simulink model "Final"  (R2025b)
settings: Solver=ode4  StartTime=0.0  StopTime=3  FixedStep=1e-5  RelTol=1e-3
values from neighbouring files (symbols this model uses):
  BAT_A = BAT    [simulink_init_params_CORRECTED.m]
  BAT_B = BAT    [simulink_init_params_CORRECTED.m]
  omega_init_cmd = SpeedRef_rpm_cmd * 2 * pi / 60    (= 314.159265359)    [simulink_init_params_CORRECTED.m]
  SpeedRef_rpm_cmd = 3000    [simulink_init_params_CORRECTED.m]
  TorqueRef_gen_Nm_cmd = -100    [simulink_init_params_CORRECTED.m]
undefined symbols (not defined in the file or in its folder): BAT, DCDC, DCLINK, FOC, FW, INV, MECH, PMSM, THERM
libraries: slpidlib x6, mcbcontrolslib x2
(part 1 of 2)
settings Model: Creator=barne  LastModifiedBy=barne

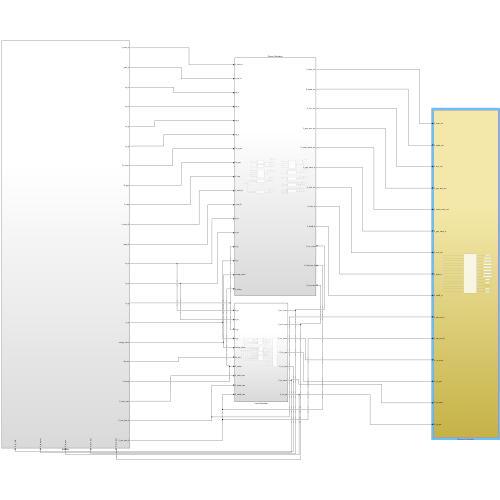
[thumbnail: Simulink's stored preview of the top-level diagram]
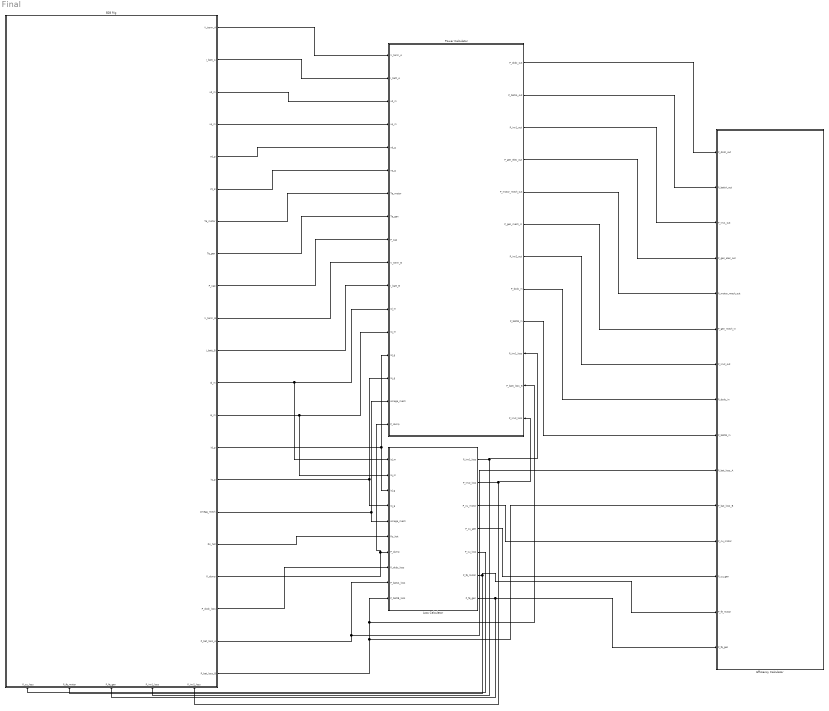
== system Final ==
  "B2B Rig " : Subsystem
      settings: PortSchema="{\"entries\":[{\"content\":{\"sides\":[{\"content\":{},\"type\":\"ConnectorPlacement.EquallySpacedRectSide\",\"uuid\":\"35d57d76-af41-41f5-b20d-811f83701aa2\"},{\"content\":{\"connectorIds\":[\"Out1\",\"Out2\",\"Out3\",\"Out4\",\"Out5\",\"Out6\",\"Out7\",\"Out8\",\"Out9\",\"Out10\",\"Out11\",\"Out12\",\"Out13\",\"Out14\",\"Out15\",\"Out16\",\"Out17\",\"Out18\",\"Out19\",\"Out20\",\"Out21\"],\"side\":\"RIGHT\"},\"type\":\"ConnectorPlacement.EquallySpacedRectSide\",\"uuid\":\"9a3983e4-5d9f-4748-b79f-80b2f2f1c763\"},{\"content\":{\"side\":\"TOP\"},\"type\":\"ConnectorPlacement.EquallySpacedRectSide\",\"uuid\":\"9f326ba3-25e1-42ff-85bf-75e4830b2979\"},{\"content\":{\"connectorIds\":[\"In1\",\"In2\",\"In3\",\"In4\",\"In5\"],\"side\":\"BOTTOM\"},\"type\":\"ConnectorPlacement.EquallySpacedRectSide\",\"uuid\":\"a03ba88c-9183-421b-aa71-4f6f8afbf457\"}]},\"type\":\"ConnectorPlacement.EquallySpacedConnector\",\"uuid\":\"4b320d25-9064-42a3-b743-e8ce904cf471\"}],\"packageUris\":[\"http://schema.mathworks.com/mf0/Connector/R2020b\"],\"version\":\"1.0\"}"
  Efficiency Calculator : Subsystem
  Loss Calculator : Subsystem
  Power Calculator : Subsystem
      settings: PortSchema="{\"entries\":[{\"content\":{\"sides\":[{\"content\":{\"connectorIds\":[\"In1\",\"In2\",\"In3\",\"In4\",\"In5\",\"In6\",\"In7\",\"In8\",\"In9\",\"In10\",\"In11\",\"In12\",\"In13\",\"In14\",\"In15\",\"In16\",\"In17\"]},\"type\":\"ConnectorPlacement.EquallySpacedRectSide\",\"uuid\":\"b3a63054-6e96-48ec-b2cd-405618c65b15\"},{\"content\":{\"connectorIds\":[\"Out1\",\"Out2\",\"Out3\",\"Out4\",\"Out5\",\"Out6\",\"Out7\",\"Out8\",\"Out9\",\"In18\",\"In19\",\"In20\"],\"side\":\"RIGHT\"},\"type\":\"ConnectorPlacement.EquallySpacedRectSide\",\"uuid\":\"702f6dd8-defa-44ea-83b1-91536885574a\"},{\"content\":{\"side\":\"TOP\"},\"type\":\"ConnectorPlacement.EquallySpacedRectSide\",\"uuid\":\"42970328-246a-4ab1-891c-aefddd02ac7d\"}]},\"type\":\"ConnectorPlacement.EquallySpacedConnector\",\"uuid\":\"4be053d2-cc40-44fc-9305-e73801c5c4b1\"}],\"packageUris\":[\"http://schema.mathworks.com/mf0/Connector/R2020b\"],\"version\":\"1.0\"}"
  wires:
  "B2B Rig "/20(P_bat_loss_A) -> Loss Calculator/9(P_battA_loss), Efficiency Calculator/10(P_bat_loss_A)
  "B2B Rig "/1(V_term_A) -> Power Calculator/1(V_term_A)
  "B2B Rig "/7(Te_motor) -> Power Calculator/7(Te_motor)
  Power Calculator/6(P_gen_mech_in) -> Efficiency Calculator/6(P_gen_mech_in)
  "B2B Rig "/19(P_dcdc_loss) -> Loss Calculator/8(P_dcdc_loss)
  "B2B Rig "/2(I_batt_A) -> Power Calculator/2(I_batt_A)
  "B2B Rig "/3(vd_m) -> Power Calculator/3("vd_m ")
  "B2B Rig "/8(Te_gen) -> Power Calculator/8(Te_gen)
  "B2B Rig "/6(vq_g) -> Power Calculator/6(vq_g)
  "B2B Rig "/4(vq_m) -> Power Calculator/4(vq_m)
  "B2B Rig "/5(vd_g) -> Power Calculator/5(vd_g)
  "B2B Rig "/10(V_term_B) -> Power Calculator/10(V_term_B)
  Power Calculator/9(P_battB_in) -> Efficiency Calculator/9(P_battB_in)
  "B2B Rig "/11(I_batt_B) -> Power Calculator/11(I_batt_B)
  "B2B Rig "/12(id_m) -> Power Calculator/12(id_m), Loss Calculator/1(id_m)
  "B2B Rig "/13(iq_m) -> Power Calculator/13(iq_m), Loss Calculator/2(iq_m)
  "B2B Rig "/14(id_g) -> Power Calculator/14(id_g), Loss Calculator/3(id_g)
  Loss Calculator/1(P_inv1_loss) -> Power Calculator/18(P_inv1_loss), "B2B Rig "/4(P_inv1_loss)
  "B2B Rig "/15(iq_g) -> Power Calculator/15(iq_g), Loss Calculator/4(iq_g)
  "B2B Rig "/16(omega_mech) -> Power Calculator/16(omega_mech), Loss Calculator/5(omega_mech)
  Power Calculator/8(P_dcdc_in) -> Efficiency Calculator/8(P_dcdc_in)
  Power Calculator/4(P_gen_elec_out) -> Efficiency Calculator/4(P_gen_elec_out)
  "B2B Rig "/17(Rs_hot) -> Loss Calculator/6(Rs_hot)
  "B2B Rig "/18(P_dump) -> Power Calculator/17(P_dump), Loss Calculator/7(P_dump)
  "B2B Rig "/21(P_bat_loss_B) -> Loss Calculator/10(P_battB_loss), Power Calculator/19(P_batt_loss_B), Efficiency Calculator/11(P_bat_loss_B)
  Power Calculator/2(P_battA_out) -> Efficiency Calculator/2(P_battA_out)
  Power Calculator/3(P_inv1_out) -> Efficiency Calculator/3(P_inv1_out)
  Power Calculator/5(P_motor_mech_out) -> Efficiency Calculator/5(P_motor_mech_out)
  Power Calculator/7(P_inv2_out) -> Efficiency Calculator/7(P_inv2_out)
  Power Calculator/1(P_dcdc_out) -> Efficiency Calculator/1(P_dcdc_out)
  "B2B Rig "/9(P_cap) -> Power Calculator/9(P_cap)
  Loss Calculator/2(P_inv2_loss) -> Power Calculator/20(P_inv2_loss), "B2B Rig "/5(P_inv2_loss)
  Loss Calculator/5(P_cu_loss) -> "B2B Rig "/1(P_cu_loss)
  Loss Calculator/3(P_cu_motor) -> Efficiency Calculator/12(P_cu_motor)
  Loss Calculator/4(P_cu_gen) -> Efficiency Calculator/13(P_cu_gen)
  Loss Calculator/6(P_fe_motor) -> Efficiency Calculator/14(P_fe_motor), "B2B Rig "/2(P_fe_motor)
  Loss Calculator/7(P_fe_gen) -> "B2B Rig "/3(P_fe_gen), Efficiency Calculator/15(P_fe_gen)

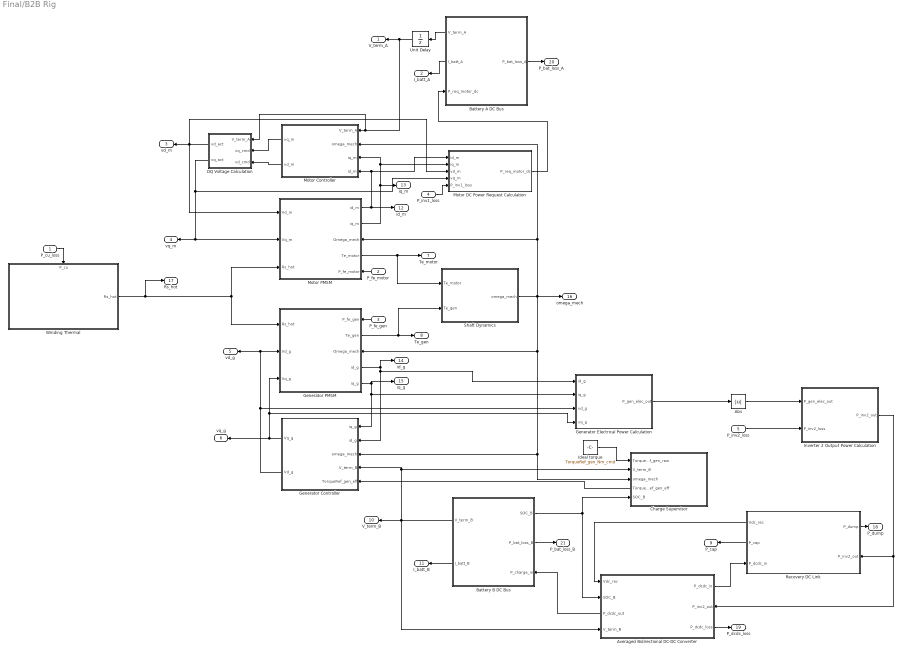
== system Final/B2B Rig  ==
  P_cu_loss : Inport
  P_fe_motor : Inport  Port=2
  P_fe_gen : Inport  Port=3
  P_inv1_loss : Inport  Port=4
  P_inv2_loss : Inport  Port=5
  Abs : Abs  SaturateOnIntegerOverflow=off
  Averaged Bidirectional DC-DC Converter : Subsystem
      settings: PortSchema="{\"entries\":[{\"content\":{\"sides\":[{\"content\":{\"connectorIds\":[\"In1\",\"In2\",\"Out3\",\"In3\"]},\"type\":\"ConnectorPlacement.EquallySpacedRectSide\",\"uuid\":\"c75c4d97-d9fe-4485-978f-a90415bcd4b0\"},{\"content\":{\"connectorIds\":[\"Out1\",\"In4\",\"Out2\"],\"side\":\"RIGHT\"},\"type\":\"ConnectorPlacement.EquallySpacedRectSide\",\"uuid\":\"ca166856-9308-4393-8aae-1a6df3904c27\"},{\"content\":{\"side\":\"TOP\"},\"type\":\"ConnectorPlacement.EquallySpacedRectSide\",\"uuid\":\"ee8baf38-1402-4df1-aabb-1ba4a360531c\"}]},\"type\":\"ConnectorPlacement.EquallySpacedConnector\",\"uuid\":\"7d2a7e48-193d-4e7a-9033-8960d9759152\"}],\"packageUris\":[\"http://schema.mathworks.com/mf0/Connector/R2020b\"],\"version\":\"1.0\"}"
  Battery A DC Bus : Subsystem
      settings: PortSchema="{\"entries\":[{\"content\":{\"sides\":[{\"content\":{\"connectorIds\":[\"Out2\",\"Out3\",\"In1\"]},\"type\":\"ConnectorPlacement.EquallySpacedRectSide\",\"uuid\":\"be2ffeb8-897f-4fb0-9a8e-cb986b650704\"},{\"content\":{\"connectorIds\":[\"Out1\"],\"side\":\"RIGHT\"},\"type\":\"ConnectorPlacement.EquallySpacedRectSide\",\"uuid\":\"a4a4824a-f919-417d-bceb-2ba105cf5ab4\"},{\"content\":{\"side\":\"TOP\"},\"type\":\"ConnectorPlacement.EquallySpacedRectSide\",\"uuid\":\"5f1b089a-09aa-462b-ad0f-8275eb166d2e\"}]},\"type\":\"ConnectorPlacement.EquallySpacedConnector\",\"uuid\":\"42065a04-5d0c-471f-9e1f-47cde4d39611\"}],\"packageUris\":[\"http://schema.mathworks.com/mf0/Connector/R2020b\"],\"version\":\"1.0\"}"
  Battery B DC Bus : Subsystem
      settings: PortSchema="{\"entries\":[{\"content\":{\"sides\":[{\"content\":{\"connectorIds\":[\"Out3\",\"Out4\"]},\"type\":\"ConnectorPlacement.EquallySpacedRectSide\",\"uuid\":\"be2ffeb8-897f-4fb0-9a8e-cb986b650704\"},{\"content\":{\"connectorIds\":[\"Out1\",\"Out2\",\"In1\"],\"side\":\"RIGHT\"},\"type\":\"ConnectorPlacement.EquallySpacedRectSide\",\"uuid\":\"a4a4824a-f919-417d-bceb-2ba105cf5ab4\"},{\"content\":{\"side\":\"TOP\"},\"type\":\"ConnectorPlacement.EquallySpacedRectSide\",\"uuid\":\"5f1b089a-09aa-462b-ad0f-8275eb166d2e\"}]},\"type\":\"ConnectorPlacement.EquallySpacedConnector\",\"uuid\":\"42065a04-5d0c-471f-9e1f-47cde4d39611\"}],\"packageUris\":[\"http://schema.mathworks.com/mf0/Connector/R2020b\"],\"version\":\"1.0\"}"
  Charge Supervisor : Subsystem
      settings: PortSchema="{\"entries\":[{\"content\":{\"sides\":[{\"content\":{\"connectorIds\":[\"In1\",\"In2\",\"In3\",\"Out1\",\"In4\"]},\"type\":\"ConnectorPlacement.EquallySpacedRectSide\",\"uuid\":\"511ba033-72f1-459a-95dc-757aaac28559\"},{\"content\":{\"side\":\"RIGHT\"},\"type\":\"ConnectorPlacement.EquallySpacedRectSide\",\"uuid\":\"14c3a67f-ee08-4dd0-a6b8-6f3110f3c251\"},{\"content\":{\"side\":\"TOP\"},\"type\":\"ConnectorPlacement.EquallySpacedRectSide\",\"uuid\":\"028d3826-294c-4b4b-bd61-9c2d945a5125\"}]},\"type\":\"ConnectorPlacement.EquallySpacedConnector\",\"uuid\":\"eacb2f62-77aa-43a8-a347-5c269c986bc2\"}],\"packageUris\":[\"http://schema.mathworks.com/mf0/Connector/R2020b\"],\"version\":\"1.0\"}"
  DQ Voltage Calculation : MATLAB Function  TreatAsAtomicUnit=on
  Generator Controller : Subsystem
  Generator Electrical Power Calculation : MATLAB Function  TreatAsAtomicUnit=on
  Generator PMSM : Subsystem
      settings: PortSchema="{\"entries\":[{\"content\":{\"sides\":[{\"content\":{\"connectorIds\":[\"In1\",\"In2\",\"In3\"]},\"type\":\"ConnectorPlacement.EquallySpacedRectSide\",\"uuid\":\"07b3d59a-f926-4a7d-ab04-b9c2d2b414a8\"},{\"content\":{\"connectorIds\":[\"In4\",\"Out1\",\"In5\",\"Out2\",\"Out3\"],\"side\":\"RIGHT\"},\"type\":\"ConnectorPlacement.EquallySpacedRectSide\",\"uuid\":\"bee2f74a-f43a-4aee-bb40-851f5cf071b9\"},{\"content\":{\"side\":\"TOP\"},\"type\":\"ConnectorPlacement.EquallySpacedRectSide\",\"uuid\":\"c59a3e1f-4ae4-432c-9c2c-e4c61d9f9d5f\"}]},\"type\":\"ConnectorPlacement.EquallySpacedConnector\",\"uuid\":\"492bf2cb-efe4-439e-9d58-c452a678f7e2\"}],\"packageUris\":[\"http://schema.mathworks.com/mf0/Connector/R2020b\"],\"version\":\"1.0\"}"
  "Ideal torque " : Constant  Value=TorqueRef_gen_Nm_cmd
  Inverter 2 Output Power Calculation : MATLAB Function  TreatAsAtomicUnit=on
  Motor Controller : Subsystem
  Motor DC Power Request Calculation : MATLAB Function  TreatAsAtomicUnit=on
  Motor PMSM : Subsystem
      settings: PortSchema="{\"entries\":[{\"content\":{\"sides\":[{\"content\":{\"connectorIds\":[\"In1\",\"In2\",\"In3\"]},\"type\":\"ConnectorPlacement.EquallySpacedRectSide\",\"uuid\":\"07b3d59a-f926-4a7d-ab04-b9c2d2b414a8\"},{\"content\":{\"connectorIds\":[\"Out1\",\"Out2\",\"In4\",\"Out3\",\"In5\"],\"side\":\"RIGHT\"},\"type\":\"ConnectorPlacement.EquallySpacedRectSide\",\"uuid\":\"bee2f74a-f43a-4aee-bb40-851f5cf071b9\"},{\"content\":{\"side\":\"TOP\"},\"type\":\"ConnectorPlacement.EquallySpacedRectSide\",\"uuid\":\"c59a3e1f-4ae4-432c-9c2c-e4c61d9f9d5f\"}]},\"type\":\"ConnectorPlacement.EquallySpacedConnector\",\"uuid\":\"492bf2cb-efe4-439e-9d58-c452a678f7e2\"}],\"packageUris\":[\"http://schema.mathworks.com/mf0/Connector/R2020b\"],\"version\":\"1.0\"}"
  Recovery DC Link : Subsystem
      settings: PortSchema="{\"entries\":[{\"content\":{\"sides\":[{\"content\":{\"connectorIds\":[\"Out2\",\"Out3\",\"In1\"]},\"type\":\"ConnectorPlacement.EquallySpacedRectSide\",\"uuid\":\"bc30b136-784e-45bb-af95-843f9a6ddb33\"},{\"content\":{\"connectorIds\":[\"Out1\",\"In2\"],\"side\":\"RIGHT\"},\"type\":\"ConnectorPlacement.EquallySpacedRectSide\",\"uuid\":\"2f565876-dfa7-4c6c-9c16-5c008dcf0872\"},{\"content\":{\"side\":\"TOP\"},\"type\":\"ConnectorPlacement.EquallySpacedRectSide\",\"uuid\":\"25b582a4-9873-4df9-8c8d-16d41c520507\"}]},\"type\":\"ConnectorPlacement.EquallySpacedConnector\",\"uuid\":\"ee427943-397a-4e08-9409-61b509181f95\"}],\"packageUris\":[\"http://schema.mathworks.com/mf0/Connector/R2020b\"],\"version\":\"1.0\"}"
  Shaft Dynamics : Subsystem
  Unit Delay : UnitDelay  InitialCondition=BAT_A.V_nom  SampleTime=FOC.Ts  HasFrameUpgradeWarning=on
  Winding Thermal : Subsystem
      settings: PortSchema="{\"entries\":[{\"content\":{\"sides\":[{\"content\":{\"connectorIds\":[\"Out1\"]},\"type\":\"ConnectorPlacement.EquallySpacedRectSide\",\"uuid\":\"4eefefd2-644d-4013-be3c-911fe82f6150\"},{\"content\":{\"side\":\"RIGHT\"},\"type\":\"ConnectorPlacement.EquallySpacedRectSide\",\"uuid\":\"de5532ad-21e1-424d-bba4-8a6bf70e2e70\"},{\"content\":{\"connectorIds\":[\"In1\"],\"side\":\"TOP\"},\"type\":\"ConnectorPlacement.EquallySpacedRectSide\",\"uuid\":\"20b811fb-5177-4825-9338-966d2d4b1cfa\"}]},\"type\":\"ConnectorPlacement.EquallySpacedConnector\",\"uuid\":\"f93ab436-6edc-4857-8a77-fc7572dced6a\"}],\"packageUris\":[\"http://schema.mathworks.com/mf0/Connector/R2020b\"],\"version\":\"1.0\"}"
  V_term_A : Outport
  I_batt_A : Outport  Port=2
  vd_m : Outport  Port=3
  vq_m : Outport  Port=4
  vd_g : Outport  Port=5
  vq_g : Outport  Port=6
  Te_motor : Outport  Port=7
  Te_gen : Outport  Port=8
  P_cap : Outport  Port=9
  V_term_B : Outport  Port=10
  I_batt_B : Outport  Port=11
  id_m : Outport  Port=12
  iq_m : Outport  Port=13
  id_g : Outport  Port=14
  iq_g : Outport  Port=15
  omega_mech : Outport  Port=16
  Rs_hot : Outport  Port=17
  P_dump : Outport  Port=18
  P_dcdc_loss : Outport  Port=19
  P_bat_loss_A : Outport  Port=20
  P_bat_loss_B : Outport  Port=21
  wires:
  Battery B DC Bus/1(SOC_B) -> Charge Supervisor/4(SOC_B), Averaged Bidirectional DC-DC Converter/2(SOC_B)
  Shaft Dynamics/1(omega_mech) -> Motor Controller/2(omega_mech), Motor PMSM/4(Omega_mech), omega_mech/1, Charge Supervisor/3(omega_mech), Generator Controller/3(omega_mech), Generator PMSM/5(Omega_mech)
  Battery B DC Bus/3(V_term_B) -> Averaged Bidirectional DC-DC Converter/3(V_term_B), V_term_B/1, Generator Controller/4(V_term_B), Charge Supervisor/2(V_term_B)
  Winding Thermal/1(Rs_hot) -> Rs_hot/1, Generator PMSM/1(Rs_hot), Motor PMSM/3(Rs_hot)
  Averaged Bidirectional DC-DC Converter/3(P_dcdc_out) -> Battery B DC Bus/1(P_charge_in)
  Motor PMSM/1(id_m) -> Motor DC Power Request Calculation/1(id_m), Motor Controller/4(id_m), id_m/1
  Generator PMSM/3(iq_g) -> iq_g/1, Generator Controller/1(iq_g), Generator Electrical Power Calculation/2(iq_g)
  Motor PMSM/2(iq_m) -> Motor Controller/3(iq_m), Motor DC Power Request Calculation/2(iq_m), iq_m/1
  Recovery DC Link/1(P_dump) -> P_dump/1
  P_cu_loss/1 -> Winding Thermal/1(P_cu)
  Recovery DC Link/2(Vdc_rec) -> Averaged Bidirectional DC-DC Converter/1(Vdc_rec)
  Battery A DC Bus/2(V_term_A) -> Unit Delay/1
  Averaged Bidirectional DC-DC Converter/1(P_dcdc_in) -> Recovery DC Link/1(P_dcdc_in)
  Generator Controller/1(Vq_g) -> Generator Electrical Power Calculation/4(vq_g), Generator PMSM/3(Vq_g), vq_g/1
  Generator Controller/2(Vd_g) -> vd_g/1, Generator PMSM/2(Vd_g), Generator Electrical Power Calculation/3(vd_g)
  Motor PMSM/3(Te_motor) -> Shaft Dynamics/1(Te_motor), Te_motor/1
  Generator PMSM/1(Te_gen) -> Shaft Dynamics/2(Te_gen), Te_gen/1
  "Ideal torque "/1 -> Charge Supervisor/1(TorqueRef_gen_raw)
  Averaged Bidirectional DC-DC Converter/2(P_dcdc_loss) -> P_dcdc_loss/1
  Battery A DC Bus/1(P_bat_loss_A) -> P_bat_loss_A/1
  Battery B DC Bus/2(P_bat_loss_B) -> P_bat_loss_B/1
  Battery B DC Bus/4(I_batt_B) -> I_batt_B/1
  Motor DC Power Request Calculation/1(P_req_motor_dc) -> Battery A DC Bus/1(P_req_motor_dc)
  Charge Supervisor/1(TorqueRef_gen_eff) -> Generator Controller/5(TorqueRef_gen_eff)
  Generator PMSM/2(id_g) -> id_g/1, Generator Electrical Power Calculation/1(id_g), Generator Controller/2(id_g)
  Generator Electrical Power Calculation/1(P_gen_elec_out) -> Abs/1
  Unit Delay/1 -> DQ Voltage Calculation/1(V_term_A), Motor Controller/1(V_term_A), V_term_A/1
  Battery A DC Bus/3(I_batt_A) -> I_batt_A/1
  P_fe_motor/1 -> Motor PMSM/5(P_fe_motor)
  Motor Controller/1(vq_m) -> DQ Voltage Calculation/2(vq_cmd)
  Motor Controller/2(vd_m) -> DQ Voltage Calculation/3(vd_cmd)
  DQ Voltage Calculation/1(vd_act) -> Motor PMSM/1(Vd_m), Motor DC Power Request Calculation/3(vd_m), vd_m/1
  DQ Voltage Calculation/2(vq_act) -> vq_m/1, Motor PMSM/2(Vq_m), Motor DC Power Request Calculation/4(vq_m)
  Recovery DC Link/3(P_cap) -> P_cap/1
  P_fe_gen/1 -> Generator PMSM/4(P_fe_gen)
  P_inv1_loss/1 -> Motor DC Power Request Calculation/5(P_inv1_loss)
  P_inv2_loss/1 -> Inverter 2 Output Power Calculation/2(P_inv2_loss)
  Abs/1 -> Inverter 2 Output Power Calculation/1(P_gen_elec_out)
  Inverter 2 Output Power Calculation/1(P_inv2_out) -> Recovery DC Link/2(P_inv2_out), Averaged Bidirectional DC-DC Converter/4(P_inv2_out)

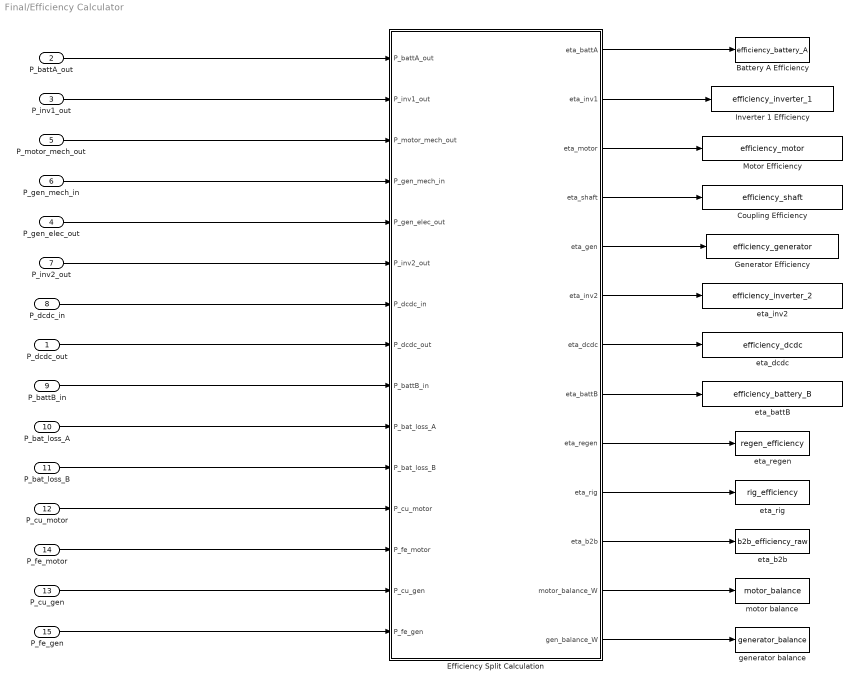
== system Final/Efficiency Calculator ==
  P_dcdc_out : Inport
  P_battA_out : Inport  Port=2
  P_inv1_out : Inport  Port=3
  P_gen_elec_out : Inport  Port=4
  P_motor_mech_out : Inport  Port=5
  P_gen_mech_in : Inport  Port=6
  P_inv2_out : Inport  Port=7
  P_dcdc_in : Inport  Port=8
  P_battB_in : Inport  Port=9
  P_bat_loss_A : Inport  Port=10
  P_bat_loss_B : Inport  Port=11
  P_cu_motor : Inport  Port=12
  P_cu_gen : Inport  Port=13
  P_fe_motor : Inport  Port=14
  P_fe_gen : Inport  Port=15
  Battery A Efficiency : ToWorkspace  VariableName=efficiency_battery_A  SaveFormat=Timeseries  SampleTime=-1
  Coupling Efficiency : ToWorkspace  VariableName=efficiency_shaft  SaveFormat=Timeseries  SampleTime=-1
  Efficiency Split Calculation : MATLAB Function  TreatAsAtomicUnit=on
  Generator Efficiency : ToWorkspace  VariableName=efficiency_generator  SaveFormat=Timeseries  SampleTime=-1
  Inverter 1 Efficiency : ToWorkspace  VariableName=efficiency_inverter_1  SaveFormat=Timeseries  SampleTime=-1
  Motor Efficiency : ToWorkspace  VariableName=efficiency_motor  SaveFormat=Timeseries  SampleTime=-1
  eta_b2b : ToWorkspace  VariableName=b2b_efficiency_raw  SaveFormat=Timeseries  SampleTime=-1
  eta_battB : ToWorkspace  VariableName=efficiency_battery_B  SaveFormat=Timeseries  SampleTime=-1
  eta_dcdc : ToWorkspace  VariableName=efficiency_dcdc  SaveFormat=Timeseries  SampleTime=-1
  eta_inv2 : ToWorkspace  VariableName=efficiency_inverter_2  SaveFormat=Timeseries  SampleTime=-1
  eta_regen : ToWorkspace  VariableName=regen_efficiency  SaveFormat=Timeseries  SampleTime=-1
  eta_rig : ToWorkspace  VariableName=rig_efficiency  SaveFormat=Timeseries  SampleTime=-1
  generator balance : ToWorkspace  VariableName=generator_balance  SaveFormat=Timeseries  SampleTime=-1
  motor balance : ToWorkspace  VariableName=motor_balance  SaveFormat=Timeseries  SampleTime=-1
  wires:
  Efficiency Split Calculation/1(eta_battA) -> Battery A Efficiency/1
  Efficiency Split Calculation/2(eta_inv1) -> Inverter 1 Efficiency/1
  Efficiency Split Calculation/3(eta_motor) -> Motor Efficiency/1
  Efficiency Split Calculation/4(eta_shaft) -> Coupling Efficiency/1
  Efficiency Split Calculation/5(eta_gen) -> Generator Efficiency/1
  Efficiency Split Calculation/6(eta_inv2) -> eta_inv2/1
  Efficiency Split Calculation/7(eta_dcdc) -> eta_dcdc/1
  Efficiency Split Calculation/8(eta_battB) -> eta_battB/1
  Efficiency Split Calculation/10(eta_rig) -> eta_rig/1
  P_inv1_out/1 -> Efficiency Split Calculation/2(P_inv1_out)
  P_motor_mech_out/1 -> Efficiency Split Calculation/3(P_motor_mech_out)
  P_gen_mech_in/1 -> Efficiency Split Calculation/4(P_gen_mech_in)
  P_gen_elec_out/1 -> Efficiency Split Calculation/5(P_gen_elec_out)
  P_dcdc_in/1 -> Efficiency Split Calculation/7(P_dcdc_in)
  P_dcdc_out/1 -> Efficiency Split Calculation/8(P_dcdc_out)
  P_battB_in/1 -> Efficiency Split Calculation/9(P_battB_in)
  P_bat_loss_A/1 -> Efficiency Split Calculation/10(P_bat_loss_A)
  P_inv2_out/1 -> Efficiency Split Calculation/6(P_inv2_out)
  P_battA_out/1 -> Efficiency Split Calculation/1(P_battA_out)
  P_bat_loss_B/1 -> Efficiency Split Calculation/11(P_bat_loss_B)
  Efficiency Split Calculation/11(eta_b2b) -> eta_b2b/1
  Efficiency Split Calculation/9(eta_regen) -> eta_regen/1
  P_cu_motor/1 -> Efficiency Split Calculation/12(P_cu_motor)
  P_cu_gen/1 -> Efficiency Split Calculation/14(P_cu_gen)
  P_fe_motor/1 -> Efficiency Split Calculation/13(P_fe_motor)
  P_fe_gen/1 -> Efficiency Split Calculation/15(P_fe_gen)
  Efficiency Split Calculation/12(motor_balance_W) -> motor balance/1
  Efficiency Split Calculation/13(gen_balance_W) -> generator balance/1

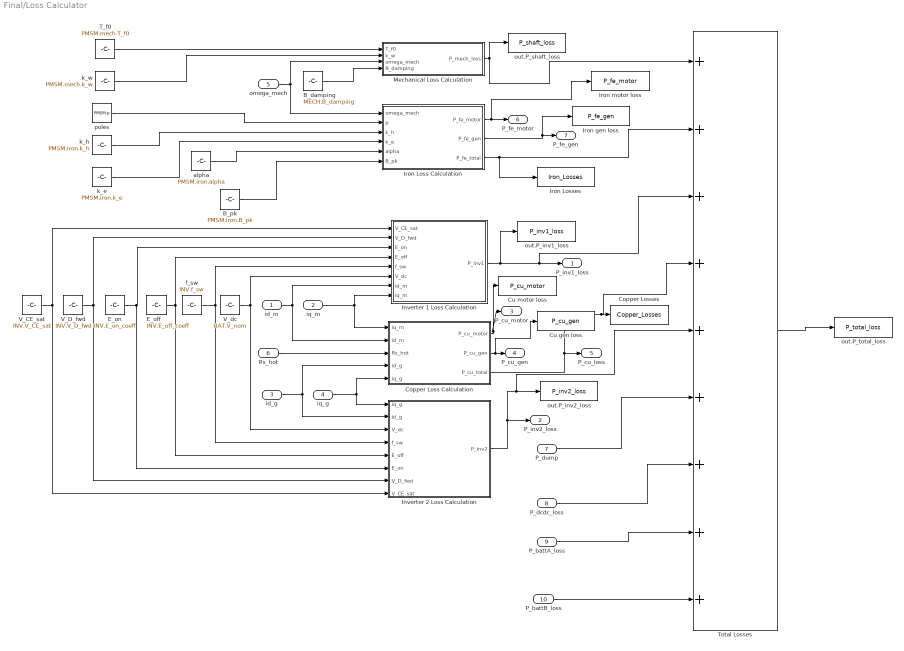
== system Final/Loss Calculator ==
  id_m : Inport
  iq_m : Inport  Port=2
  id_g : Inport  Port=3
  iq_g : Inport  Port=4
  omega_mech : Inport  Port=5
  Rs_hot : Inport  Port=6
  P_dump : Inport  Port=7
  P_dcdc_loss : Inport  Port=8
  P_battA_loss : Inport  Port=9
  P_battB_loss : Inport  Port=10
  " out.P_inv1_loss" : ToWorkspace  VariableName=P_inv1_loss  SaveFormat=Timeseries  SampleTime=-1
  B_damping : Constant  Value=MECH.B_damping
  B_pk : Constant  Value=PMSM.iron.B_pk
  Copper Loss Calculation : MATLAB Function  TreatAsAtomicUnit=on
  Copper Losses : ToWorkspace  VariableName=Copper_Losses  SaveFormat=Timeseries  SampleTime=-1
  Cu gen loss : ToWorkspace  VariableName=P_cu_gen  SaveFormat=Timeseries  SampleTime=-1
  Cu motor loss : ToWorkspace  VariableName=P_cu_motor  SaveFormat=Timeseries  SampleTime=-1
  E_off : Constant  Value=INV.E_off_coeff
  E_on : Constant  Value=INV.E_on_coeff
  Inverter 1 Loss Calculation : MATLAB Function  TreatAsAtomicUnit=on
  Inverter 2 Loss Calculation : MATLAB Function  TreatAsAtomicUnit=on
  Iron Loss Calculation : MATLAB Function  TreatAsAtomicUnit=on
  Iron Losses : ToWorkspace  VariableName=Iron_Losses  SaveFormat=Timeseries  SampleTime=-1
  Iron gen loss : ToWorkspace  VariableName=P_fe_gen  SaveFormat=Timeseries  SampleTime=-1
  Iron motor loss : ToWorkspace  VariableName=P_fe_motor  SaveFormat=Timeseries  SampleTime=-1
  Mechanical Loss Calculation : MATLAB Function  TreatAsAtomicUnit=on
  T_f0 : Constant  Value=PMSM.mech.T_f0
  Total Losses : Sum  Inputs=+++++++++
  V_CE_sat : Constant  Value=INV.V_CE_sat
  V_D_fwd : Constant  Value=INV.V_D_fwd
  V_dc : Constant  Value=BAT.V_nom
  alpha : Constant  Value=PMSM.iron.alpha
  f_sw : Constant  Value=INV.f_sw
  k_e : Constant  Value=PMSM.iron.k_e
  k_h : Constant  Value=PMSM.iron.k_h
  k_w : Constant  Value=PMSM.mech.k_w
  out.P_inv2_loss : ToWorkspace  VariableName=P_inv2_loss  SaveFormat=Timeseries  SampleTime=-1
  out.P_shaft_loss : ToWorkspace  VariableName=P_shaft_loss  SaveFormat=Timeseries  SampleTime=-1
  out.P_total_loss : ToWorkspace  VariableName=P_total_loss  SaveFormat=Timeseries  SampleTime=-1
  poles : Constant  Value=PMSM.p
  P_inv1_loss : Outport
  P_inv2_loss : Outport  Port=2
  P_cu_motor : Outport  Port=3
  P_cu_gen : Outport  Port=4
  P_cu_loss : Outport  Port=5
  P_fe_motor : Outport  Port=6
  P_fe_gen : Outport  Port=7
  wires:
  iq_g/1 -> Inverter 2 Loss Calculation/1(iq_g), Copper Loss Calculation/5(iq_g)
  id_g/1 -> Copper Loss Calculation/4(id_g), Inverter 2 Loss Calculation/2(id_g)
  iq_m/1 -> Inverter 1 Loss Calculation/8(iq_m), Copper Loss Calculation/1(iq_m)
  id_m/1 -> Copper Loss Calculation/2(id_m), Inverter 1 Loss Calculation/7(id_m)
  omega_mech/1 -> Mechanical Loss Calculation/3(omega_mech), Iron Loss Calculation/1(omega_mech)
  Inverter 1 Loss Calculation/1(P_inv1) -> " out.P_inv1_loss"/1, Total Losses/3, P_inv1_loss/1
  Inverter 2 Loss Calculation/1(P_inv2) -> Total Losses/5, out.P_inv2_loss/1, P_inv2_loss/1
  Mechanical Loss Calculation/1(P_mech_loss) -> Total Losses/1, out.P_shaft_loss/1
  V_CE_sat/1 -> Inverter 2 Loss Calculation/8(V_CE_sat), Inverter 1 Loss Calculation/1(V_CE_sat)
  V_D_fwd/1 -> Inverter 2 Loss Calculation/7(V_D_fwd), Inverter 1 Loss Calculation/2(V_D_fwd)
  E_on/1 -> Inverter 2 Loss Calculation/6(E_on), Inverter 1 Loss Calculation/3(E_on)
  E_off/1 -> Inverter 2 Loss Calculation/5(E_off), Inverter 1 Loss Calculation/4(E_off)
  f_sw/1 -> Inverter 2 Loss Calculation/4(f_sw), Inverter 1 Loss Calculation/5(f_sw)
  V_dc/1 -> Inverter 2 Loss Calculation/3(V_dc), Inverter 1 Loss Calculation/6(V_dc)
  Rs_hot/1 -> Copper Loss Calculation/3(Rs_hot)
  T_f0/1 -> Mechanical Loss Calculation/1(T_f0)
  k_w/1 -> Mechanical Loss Calculation/2(k_w)
  poles/1 -> Iron Loss Calculation/2(p)
  k_h/1 -> Iron Loss Calculation/3(k_h)
  k_e/1 -> Iron Loss Calculation/4(k_e)
  alpha/1 -> Iron Loss Calculation/5(alpha)
  B_pk/1 -> Iron Loss Calculation/6(B_pk)
  B_damping/1 -> Mechanical Loss Calculation/4(B_damping)
  P_dump/1 -> Total Losses/6
  P_dcdc_loss/1 -> Total Losses/7
  Total Losses/1 -> out.P_total_loss/1
  Copper Loss Calculation/3(P_cu_total) -> Total Losses/4, Copper Losses/1, P_cu_loss/1
  Copper Loss Calculation/1(P_cu_motor) -> Cu motor loss/1, P_cu_motor/1
  Copper Loss Calculation/2(P_cu_gen) -> Cu gen loss/1, P_cu_gen/1
  Iron Loss Calculation/3(P_fe_total) -> Total Losses/2, Iron Losses/1
  Iron Loss Calculation/1(P_fe_motor) -> Iron motor loss/1, P_fe_motor/1
  Iron Loss Calculation/2(P_fe_gen) -> Iron gen loss/1, P_fe_gen/1
  P_battA_loss/1 -> Total Losses/8
  P_battB_loss/1 -> Total Losses/9

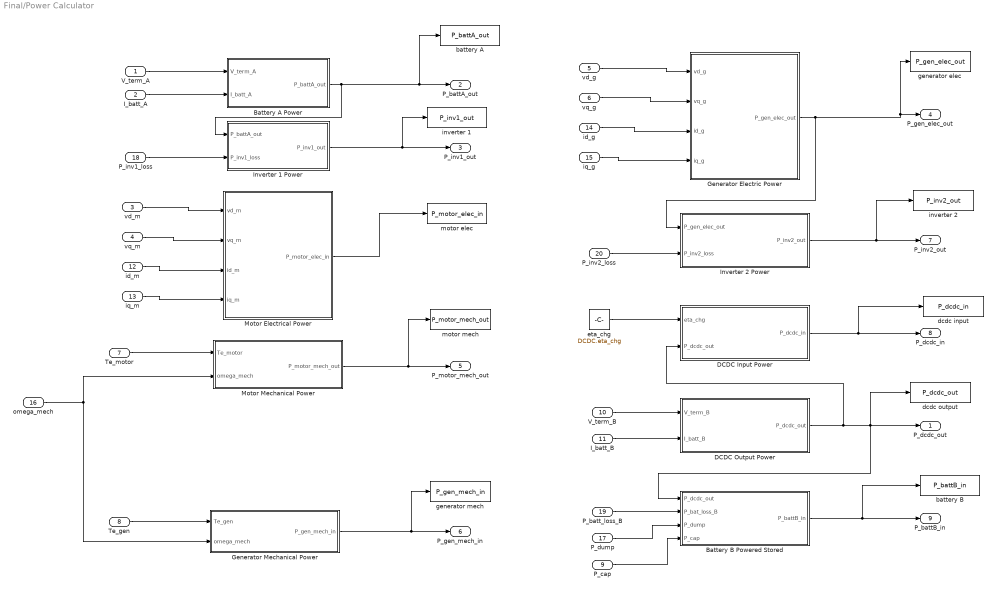
== system Final/Power Calculator ==
  V_term_A : Inport
  I_batt_A : Inport  Port=2
  "vd_m " : Inport  Port=3
  vq_m : Inport  Port=4
  vd_g : Inport  Port=5
  vq_g : Inport  Port=6
  Te_motor : Inport  Port=7
  Te_gen : Inport  Port=8
  P_cap : Inport  Port=9
  V_term_B : Inport  Port=10
  I_batt_B : Inport  Port=11
  id_m : Inport  Port=12
  iq_m : Inport  Port=13
  id_g : Inport  Port=14
  iq_g : Inport  Port=15
  omega_mech : Inport  Port=16
  P_dump : Inport  Port=17
  P_inv1_loss : Inport  Port=18
  P_batt_loss_B : Inport  Port=19
  P_inv2_loss : Inport  Port=20
  "Battery A Power " : MATLAB Function  TreatAsAtomicUnit=on
  Battery B Powered Stored : MATLAB Function  TreatAsAtomicUnit=on
  DCDC Input Power : MATLAB Function  TreatAsAtomicUnit=on
  DCDC Output Power : MATLAB Function  TreatAsAtomicUnit=on
  Generator Electric Power : MATLAB Function  TreatAsAtomicUnit=on
  Generator Mechanical Power : MATLAB Function  TreatAsAtomicUnit=on
  Inverter 1 Power : MATLAB Function  TreatAsAtomicUnit=on
  Inverter 2 Power : MATLAB Function  TreatAsAtomicUnit=on
  Motor Electrical Power : MATLAB Function  TreatAsAtomicUnit=on
  Motor Mechanical Power : MATLAB Function  TreatAsAtomicUnit=on
  battery A : ToWorkspace  VariableName=P_battA_out  SaveFormat=Timeseries  SampleTime=-1
  battery B : ToWorkspace  VariableName=P_battB_in  SaveFormat=Timeseries  SampleTime=-1
  dcdc input : ToWorkspace  VariableName=P_dcdc_in  SaveFormat=Timeseries  SampleTime=-1
  dcdc output : ToWorkspace  VariableName=P_dcdc_out  SaveFormat=Timeseries  SampleTime=-1
  eta_chg : Constant  Value=DCDC.eta_chg
  generator elec : ToWorkspace  VariableName=P_gen_elec_out  SaveFormat=Timeseries  SampleTime=-1
  generator mech : ToWorkspace  VariableName=P_gen_mech_in  SaveFormat=Timeseries  SampleTime=-1
  inverter 1 : ToWorkspace  VariableName=P_inv1_out  SaveFormat=Timeseries  SampleTime=-1
  inverter 2 : ToWorkspace  VariableName=P_inv2_out  SaveFormat=Timeseries  SampleTime=-1
  motor elec : ToWorkspace  VariableName=P_motor_elec_in  SaveFormat=Timeseries  SampleTime=-1
  motor mech : ToWorkspace  VariableName=P_motor_mech_out  SaveFormat=Timeseries  SampleTime=-1
  P_dcdc_out : Outport
  P_battA_out : Outport  Port=2
  P_inv1_out : Outport  Port=3
  P_gen_elec_out : Outport  Port=4
  P_motor_mech_out : Outport  Port=5
  P_gen_mech_in : Outport  Port=6
  P_inv2_out : Outport  Port=7
  P_dcdc_in : Outport  Port=8
  P_battB_in : Outport  Port=9
  wires:
  V_term_A/1 -> "Battery A Power "/1(V_term_A)
  I_batt_A/1 -> "Battery A Power "/2(I_batt_A)
  "Battery A Power "/1(P_battA_out) -> Inverter 1 Power/1(P_battA_out), battery A/1, P_battA_out/1
  Inverter 1 Power/1(P_inv1_out) -> inverter 1/1, P_inv1_out/1
  "vd_m "/1 -> Motor Electrical Power/1(vd_m)
  vq_m/1 -> Motor Electrical Power/2(vq_m)
  id_m/1 -> Motor Electrical Power/3(id_m)
  iq_m/1 -> Motor Electrical Power/4(iq_m)
  Motor Electrical Power/1(P_motor_elec_in) -> motor elec/1
  iq_g/1 -> Generator Electric Power/4(iq_g)
  vq_g/1 -> Generator Electric Power/2(vq_g)
  id_g/1 -> Generator Electric Power/3(id_g)
  vd_g/1 -> Generator Electric Power/1(vd_g)
  Generator Electric Power/1(P_gen_elec_out) -> generator elec/1, P_gen_elec_out/1, Inverter 2 Power/1(P_gen_elec_out)
  Te_motor/1 -> Motor Mechanical Power/1(Te_motor)
  omega_mech/1 -> Motor Mechanical Power/2(omega_mech), Generator Mechanical Power/2(omega_mech)
  Motor Mechanical Power/1(P_motor_mech_out) -> motor mech/1, P_motor_mech_out/1
  Te_gen/1 -> Generator Mechanical Power/1(Te_gen)
  Generator Mechanical Power/1(P_gen_mech_in) -> generator mech/1, P_gen_mech_in/1
  V_term_B/1 -> DCDC Output Power/1(V_term_B)
  Inverter 2 Power/1(P_inv2_out) -> inverter 2/1, P_inv2_out/1
  DCDC Input Power/1(P_dcdc_in) -> dcdc input/1, P_dcdc_in/1
  DCDC Output Power/1(P_dcdc_out) -> DCDC Input Power/2(P_dcdc_out), Battery B Powered Stored/1(P_dcdc_out), P_dcdc_out/1, dcdc output/1
  I_batt_B/1 -> DCDC Output Power/2(I_batt_B)
  Battery B Powered Stored/1(P_battB_in) -> battery B/1, P_battB_in/1
  P_inv1_loss/1 -> Inverter 1 Power/2(P_inv1_loss)
  P_batt_loss_B/1 -> Battery B Powered Stored/2(P_bat_loss_B)
  eta_chg/1 -> DCDC Input Power/1(eta_chg)
  P_inv2_loss/1 -> Inverter 2 Power/2(P_inv2_loss)
  P_dump/1 -> Battery B Powered Stored/3(P_dump)
  P_cap/1 -> Battery B Powered Stored/4(P_cap)

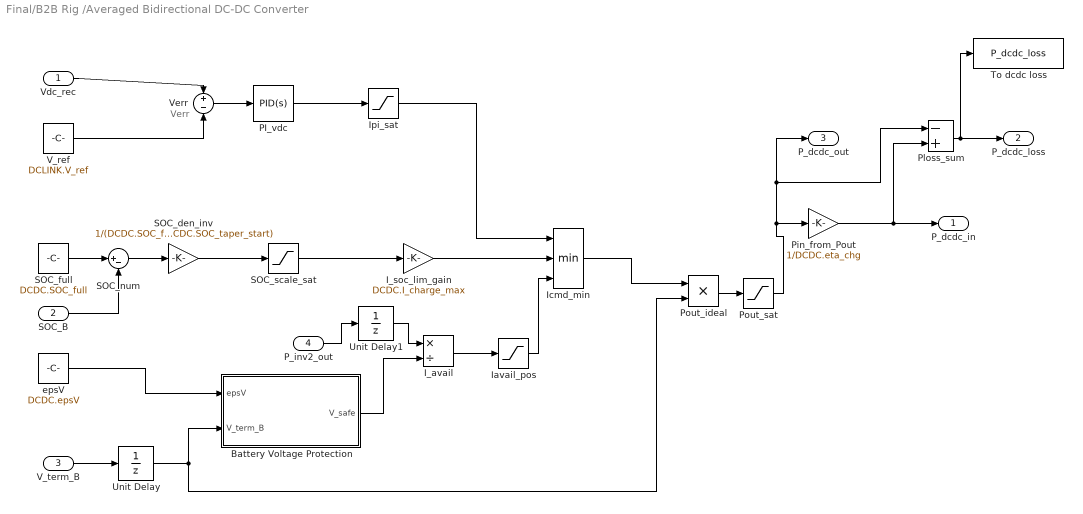
== system Final/B2B Rig /Averaged Bidirectional DC-DC Converter ==
  note: Verr
  Vdc_rec : Inport
  SOC_B : Inport  Port=2
  V_term_B : Inport  Port=3
  P_inv2_out : Inport  Port=4
  Battery Voltage Protection : MATLAB Function  TreatAsAtomicUnit=on
  I_avail : Product  Inputs=*/
  I_soc_lim_gain : Gain  Gain=DCDC.I_charge_max
  Iavail_pos : Saturate  UpperLimit=DCDC.I_charge_max  LowerLimit=0
  Icmd_min : MinMax  Inputs=3
  Ipi_sat : Saturate  UpperLimit=DCDC.I_charge_max  LowerLimit=0
  PI_vdc : slpidlib/PID Controller  Controller=PID  Form=Parallel  TimeDomain=Continuous-time  UseExternalTs=off  SampleTime=-1  IntegratorMethod=Forward Euler  FilterMethod=Forward Euler  ControllerParametersSource=internal  P=DCDC.Kp_v  I=DCDC.Ki_v  UseKiTs=off  D=0  UseExternalDerivativeSource=off  N=100  UseFilter=on  TunerSelectOption=Transfer Function Based (PID Tuner App)  InitialConditionSource=internal  InitialConditionForIntegrator=0  InitialConditionForFilter=0  DifferentiatorICPrevScaledInput=0  ExternalReset=none  TrackingMode=off  Kt=1  LimitOutput=off  SatLimitsSource=internal  UpperSaturationLimit=inf  LowerSaturationLimit=-inf  LinearizeAsGain=on  AntiWindupMode=none  Kb=1  LimitIntegrator=off  UpperIntegratorSaturationLimit=inf  LowerIntegratorSaturationLimit=-inf  POutMin=[]  POutMax=[]  IOutMin=[]  IOutMax=[]  DOutMin=[]  DOutMax=[]  NOutMin=[]  NOutMax=[]  SumOutMin=[]  SumOutMax=[]  SaturationOutMin=[]  SaturationOutMax=[]  PParamMin=[]  PParamMax=[]  IParamMin=[]  IParamMax=[]  DParamMin=[]  DParamMax=[]  NParamMin=[]  NParamMax=[]  KbParamMin=[]  KbParamMax=[]  KtParamMin=[]  KtParamMax=[]  KbOutMin=[]  KbOutMax=[]  KtOutMin=[]  KtOutMax=[]  IntegratorOutMin=[]  IntegratorOutMax=[]  FilterOutMin=[]  FilterOutMax=[]  SumI1OutMin=[]  SumI1OutMax=[]  SumI2OutMin=[]  SumI2OutMax=[]  SumI3OutMin=[]  SumI3OutMax=[]  SumI4OutMin=[]  SumI4OutMax=[]  SumDOutMin=[]  SumDOutMax=[]  DifferentiatorOutMin=[]  DifferentiatorOutMax=[]  FilterDiffOutCoefMin=[]  FilterDiffOutCoefMax=[]  ReciprocalOutMin=[]  ReciprocalOutMax=[]  SumDenOutMin=[]  SumDenOutMax=[]  SumNumOutMin=[]  SumNumOutMax=[]  DivideOutMin=[]  DivideOutMax=[]  UdiffTsProdOutMin=[]  UdiffTsProdOutMax=[]  NTsProdOutMin=[]  NTsProdOutMax=[]  UintegralTsProdOutMin=[]  UintegralTsProdOutMax=[]  UngainTsProdOutMin=[]  UngainTsProdOutMax=[]  ClampingZeroOutDataTypeStr=Inherit: Inherit via back propagation  ClampingZeroOutMin=[]  ClampingZeroOutMax=[]  FilterDenConstantOutDataTypeStr=Inherit: Inherit via back propagation  FilterDenConstantOutMin=[]  FilterDenConstantOutMax=[]  PCopyOutDataTypeStr=Inherit: Inherit via back propagation  PCopyOutMin=[]  PCopyOutMax=[]  NCopyOutDataTypeStr=Inherit: Inherit via back propagation  NCopyOutMin=[]  NCopyOutMax=[]  IntegratorContinuousStateAttributes=''  IntegratorStateMustResolveToSignalObject=off  IntegratorRTWStateStorageClass=Auto  FilterContinuousStateAttributes=''  FilterStateMustResolveToSignalObject=off  FilterRTWStateStorageClass=Auto  ParallelPVariant=InternalParameters  IdealPVariant=Disabled  IVariant=InternalParameters  DVariant=InternalParameters  IntegratorVariant=Continuous  SatVariant=Disabled  AWVariant=Passthrough  PCopyVariant=Disabled  TRVariant=Disabled  FdbkBlocksVariant=Forward  IdealPFdbkVariant=Disabled  SatFdbkVariant=Disabled  DerivativeFilterVariant=ContFilter  NVariant=InternalParameters  NCopyVariant=Disabled  FilterICVariant=InternalICsFilter  IntegratorICVariant=InternalICs  ExternalResetVariant=Disabled  TRSumVariant=Passthrough  SumFdbkVariant=Disabled  SumVariant=Sum_PID  TsampFilterVariant=InternalTs  TsampNgainVariant=Passthrough  TsampIntegralVariant=Disabled_SignalSpec  ExternalSaturationOutDataTypeStr=Inherit: Same as second input  DerivativeSourceVariant=ErrorSignal  PreIntVariant=InternalPreInt
  Pin_from_Pout : Gain  Gain=1/DCDC.eta_chg
  Ploss_sum : Sum  Inputs=-+
  Pout_ideal : Product
  Pout_sat : Saturate  UpperLimit=DCDC.P_max  LowerLimit=0
  SOC_den_inv : Gain  Gain=1/(DCDC.SOC_full-DCDC.SOC_taper_start)
  SOC_full : Constant  Value=DCDC.SOC_full
  SOC_num : Sum  Inputs=|+-
  SOC_scale_sat : Saturate  UpperLimit=1  LowerLimit=0
  To dcdc loss : ToWorkspace  VariableName=P_dcdc_loss  SaveFormat=Timeseries  SampleTime=-1
  Unit Delay : UnitDelay  InitialCondition=BAT_B.V_nom  SampleTime=FOC.Ts  HasFrameUpgradeWarning=on
  Unit Delay1 : UnitDelay  SampleTime=FOC.Ts  HasFrameUpgradeWarning=on
  V_ref : Constant  Value=DCLINK.V_ref
  Verr : Sum  Inputs=+-
  epsV : Constant  Value=DCDC.epsV
  P_dcdc_in : Outport
  P_dcdc_loss : Outport  Port=2
  P_dcdc_out : Outport  Port=3
  wires:
  Vdc_rec/1 -> Verr/1
  V_ref/1 -> Verr/2
  SOC_B/1 -> SOC_num/2
  SOC_full/1 -> SOC_num/1
  SOC_num/1 -> SOC_den_inv/1
  SOC_den_inv/1 -> SOC_scale_sat/1
  SOC_scale_sat/1 -> I_soc_lim_gain/1
  Battery Voltage Protection/1(V_safe) -> I_avail/2
  Ipi_sat/1 -> Icmd_min/1
  I_soc_lim_gain/1 -> Icmd_min/2
  Icmd_min/1 -> Pout_ideal/1
  Pout_ideal/1 -> Pout_sat/1
  Pin_from_Pout/1 -> Ploss_sum/2, P_dcdc_in/1
  Pout_sat/1 -> P_dcdc_out/1, Ploss_sum/1, Pin_from_Pout/1
  Ploss_sum/1 -> P_dcdc_loss/1, To dcdc loss/1
  V_term_B/1 -> Unit Delay/1
  Verr/1 -> PI_vdc/1
  PI_vdc/1 -> Ipi_sat/1
  Iavail_pos/1 -> Icmd_min/3
  epsV/1 -> Battery Voltage Protection/1(epsV)
  I_avail/1 -> Iavail_pos/1
  Unit Delay/1 -> Battery Voltage Protection/2(V_term_B), Pout_ideal/2
  Unit Delay1/1 -> I_avail/1
  P_inv2_out/1 -> Unit Delay1/1

== system Final/B2B Rig /Battery A DC Bus ==
  P_req_motor_dc : Inport
  Abs : Abs  SaturateOnIntegerOverflow=off
  Battery A : MATLAB Function  TreatAsAtomicUnit=on
  Battery A Current : ToWorkspace  VariableName=BattA_current  SaveFormat=Timeseries  SampleTime=-1
  C_Ah : Constant  Value=BAT.C_Ah
  R_init : Constant  Value=BAT.R_int
  SOC integrator : Integrator  InitialCondition=BAT.SOC_init  LimitOutput=on  UpperSaturationLimit=1  LowerSaturationLimit=0
  Scope : Scope
      settings: ActiveDisplayYMinimum=137427.72961862828  ActiveDisplayYMaximum=137478.10411644873
  V_max : Constant  Value=BAT.V_max
  V_min : Constant  Value=BAT.V_min
  out.P_batA_loss : ToWorkspace  VariableName=P_batA_loss  SaveFormat=Timeseries  SampleTime=-1
  P_bat_loss_A : Outport
  V_term_A : Outport  Port=2
  I_batt_A : Outport  Port=3
  wires:
  P_req_motor_dc/1 -> Abs/1
  V_max/1 -> Battery A/2(V_max)
  V_min/1 -> Battery A/3(V_min)
  R_init/1 -> Battery A/4(R_int)
  C_Ah/1 -> Battery A/5(C_Ah)
  SOC integrator/1 -> Battery A/6(SOC_A)
  Battery A/3(I_batt_A) -> Battery A Current/1, I_batt_A/1
  Abs/1 -> Battery A/1(P_req_motor_dc)
  Battery A/5(dSOC_dt) -> SOC integrator/1
  Battery A/1(V_term_A) -> V_term_A/1
  Battery A/2(P_bat_loss_A) -> out.P_batA_loss/1, P_bat_loss_A/1
  Battery A/4(P_battA_max) -> Scope/1

== system Final/B2B Rig /Battery B DC Bus ==
  P_charge_in : Inport
  Abs : Abs  SaturateOnIntegerOverflow=off
  Battery B : MATLAB Function  TreatAsAtomicUnit=on
  Battery B Current : ToWorkspace  VariableName=BattB_current  SaveFormat=Timeseries  SampleTime=-1
  C_Ah : Constant  Value=BAT.C_Ah
  I_regen_max : Constant  Value=BAT.I_regen_max
  R_init : Constant  Value=BAT.R_int
  SOC integrator : Integrator  InitialCondition=BAT_B.SOC_init  LimitOutput=on  UpperSaturationLimit=1  LowerSaturationLimit=0
  V_max : Constant  Value=BAT.V_max
  V_min : Constant  Value=BAT.V_min
  out.P_batB_loss : ToWorkspace  VariableName=P_batB_loss  SaveFormat=Timeseries  SampleTime=-1
  SOC_B : Outport
  P_bat_loss_B : Outport  Port=2
  V_term_B : Outport  Port=3
  I_batt_B : Outport  Port=4
  wires:
  P_charge_in/1 -> Abs/1
  SOC integrator/1 -> Battery B/7(SOC_B), SOC_B/1
  Battery B/4(dSOC_dt) -> SOC integrator/1
  Battery B/3(I_batt_B) -> Battery B Current/1, I_batt_B/1
  Battery B/2(P_bat_loss) -> out.P_batB_loss/1, P_bat_loss_B/1
  Battery B/1(V_term_B) -> V_term_B/1
  Abs/1 -> Battery B/1(P_charge_dc)
  V_max/1 -> Battery B/2(V_max)
  V_min/1 -> Battery B/3(V_min)
  R_init/1 -> Battery B/4(R_int)
  C_Ah/1 -> Battery B/5(C_Ah)
  I_regen_max/1 -> Battery B/6(I_charge_max)

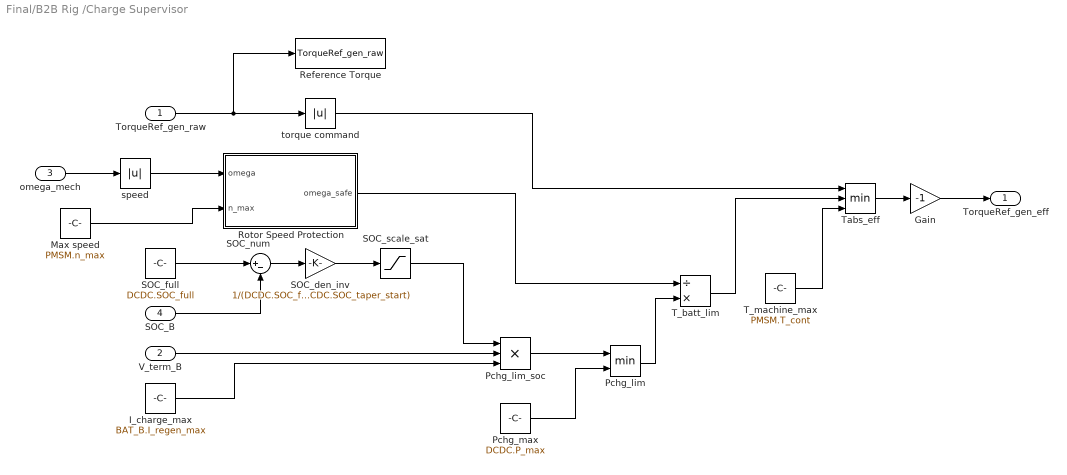
== system Final/B2B Rig /Charge Supervisor ==
  TorqueRef_gen_raw : Inport
  V_term_B : Inport  Port=2
  omega_mech : Inport  Port=3
  SOC_B : Inport  Port=4
  Gain : Gain  Gain=-1
  I_charge_max : Constant  Value=BAT_B.I_regen_max
  Max speed : Constant  Value=PMSM.n_max
  Pchg_lim : MinMax  Inputs=2
  Pchg_lim_soc : Product  Inputs=3
  Pchg_max : Constant  Value=DCDC.P_max
  Reference Torque : ToWorkspace  VariableName=TorqueRef_gen_raw  SaveFormat=Timeseries  SampleTime=-1
  Rotor Speed Protection : MATLAB Function  TreatAsAtomicUnit=on
  SOC_den_inv : Gain  Gain=1/(DCDC.SOC_full-DCDC.SOC_taper_start)
  SOC_full : Constant  Value=DCDC.SOC_full
  SOC_num : Sum  Inputs=|+-
  SOC_scale_sat : Saturate  UpperLimit=1  LowerLimit=0
  T_batt_lim : Product  Inputs=/*
  T_machine_max : Constant  Value=PMSM.T_cont
  Tabs_eff : MinMax  Inputs=3
  speed : Abs  SaturateOnIntegerOverflow=off
  torque command : Abs  SaturateOnIntegerOverflow=off
  TorqueRef_gen_eff : Outport
  wires:
  TorqueRef_gen_raw/1 -> Reference Torque/1, torque command/1
  omega_mech/1 -> speed/1
  SOC_full/1 -> SOC_num/1
  SOC_B/1 -> SOC_num/2
  SOC_num/1 -> SOC_den_inv/1
  SOC_den_inv/1 -> SOC_scale_sat/1
  I_charge_max/1 -> Pchg_lim_soc/3
  V_term_B/1 -> Pchg_lim_soc/2
  SOC_scale_sat/1 -> Pchg_lim_soc/1
  Pchg_lim_soc/1 -> Pchg_lim/1
  Pchg_max/1 -> Pchg_lim/2
  Rotor Speed Protection/1(omega_safe) -> T_batt_lim/1
  Pchg_lim/1 -> T_batt_lim/2
  torque command/1 -> Tabs_eff/1
  T_batt_lim/1 -> Tabs_eff/2
  T_machine_max/1 -> Tabs_eff/3
  Tabs_eff/1 -> Gain/1
  Gain/1 -> TorqueRef_gen_eff/1
  speed/1 -> Rotor Speed Protection/1(omega)
  Max speed/1 -> Rotor Speed Protection/2(n_max)

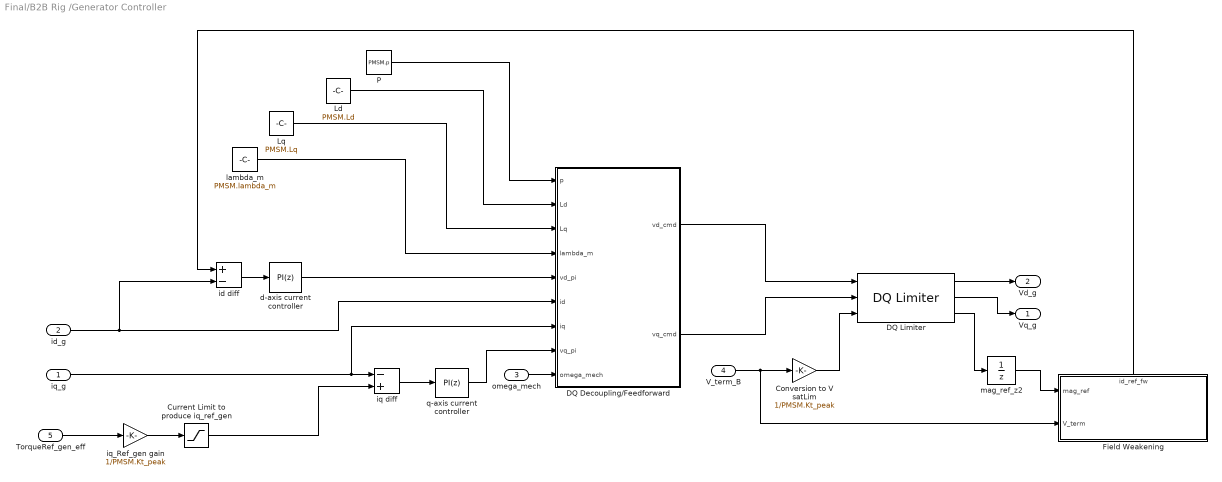
== system Final/B2B Rig /Generator Controller ==
  iq_g : Inport
  id_g : Inport  Port=2
  omega_mech : Inport  Port=3
  V_term_B : Inport  Port=4
  TorqueRef_gen_eff : Inport  Port=5
  Conversion to V satLim : Gain  Gain=1/PMSM.Kt_peak
  Current Limit to produce iq_ref_gen : Saturate  UpperLimit=466.7  LowerLimit=-466.7
  DQ Decoupling/Feedforward : MATLAB Function  TreatAsAtomicUnit=on
  DQ Limiter : mcbcontrolslib/DQ Limiter  satMethodInputType=Specify via dialog  satMethodSelected=D-Q equivalence  satLimitInputType=Input port  Vmax=153
      settings: LibrarySourceBlock=mcblib/Controls/Control Reference/DQ Limiter
  Field Weakening : Subsystem
      settings: PortSchema="{\"entries\":[{\"content\":{\"sides\":[{\"content\":{\"connectorIds\":[\"In1\",\"In2\"]},\"type\":\"ConnectorPlacement.EquallySpacedRectSide\",\"uuid\":\"203a0201-c6d3-4021-9e02-f3e52e0315c3\"},{\"content\":{\"side\":\"RIGHT\"},\"type\":\"ConnectorPlacement.EquallySpacedRectSide\",\"uuid\":\"dc29f0d6-36ca-40be-93a9-96ff6b1d1e1c\"},{\"content\":{\"connectorIds\":[\"Out1\"],\"side\":\"TOP\"},\"type\":\"ConnectorPlacement.EquallySpacedRectSide\",\"uuid\":\"ca3e0a02-f9af-4c90-ae20-302966c67b10\"}]},\"type\":\"ConnectorPlacement.EquallySpacedConnector\",\"uuid\":\"9d944e2c-da2e-448a-8f6b-8a0454a994f1\"}],\"packageUris\":[\"http://schema.mathworks.com/mf0/Connector/R2020b\"],\"version\":\"1.0\"}"
  Ld : Constant  Value=PMSM.Ld
  Lq : Constant  Value=PMSM.Lq
  P : Constant  Value=PMSM.p
  d-axis current controller : slpidlib/PID Controller  Controller=PI  Form=Parallel  TimeDomain=Discrete-time  UseExternalTs=off  SampleTime=FOC.Ts  IntegratorMethod=Forward Euler  FilterMethod=Forward Euler  ControllerParametersSource=internal  P=FOC.Kp_id  I=FOC.Ki_id  UseKiTs=off  D=0  UseExternalDerivativeSource=off  N=100  UseFilter=on  TunerSelectOption=Transfer Function Based (PID Tuner App)  InitialConditionSource=internal  InitialConditionForIntegrator=0  InitialConditionForFilter=0  DifferentiatorICPrevScaledInput=0  ExternalReset=none  TrackingMode=off  Kt=1  LimitOutput=on  SatLimitsSource=internal  UpperSaturationLimit=BAT.V_nom/sqrt(3)  LowerSaturationLimit=-BAT.V_nom/sqrt(3)  LinearizeAsGain=off  AntiWindupMode=clamping  Kb=1  LimitIntegrator=off  UpperIntegratorSaturationLimit=inf  LowerIntegratorSaturationLimit=-inf  POutMin=[]  POutMax=[]  IOutMin=[]  IOutMax=[]  DOutMin=[]  DOutMax=[]  NOutMin=[]  NOutMax=[]  SumOutMin=[]  SumOutMax=[]  SaturationOutMin=[]  SaturationOutMax=[]  PParamMin=[]  PParamMax=[]  IParamMin=[]  IParamMax=[]  DParamMin=[]  DParamMax=[]  NParamMin=[]  NParamMax=[]  KbParamMin=[]  KbParamMax=[]  KtParamMin=[]  KtParamMax=[]  KbOutMin=[]  KbOutMax=[]  KtOutMin=[]  KtOutMax=[]  IntegratorOutMin=[]  IntegratorOutMax=[]  FilterOutMin=[]  FilterOutMax=[]  SumI1OutMin=[]  SumI1OutMax=[]  SumI2OutMin=[]  SumI2OutMax=[]  SumI3OutMin=[]  SumI3OutMax=[]  SumI4OutMin=[]  SumI4OutMax=[]  SumDOutMin=[]  SumDOutMax=[]  DifferentiatorOutMin=[]  DifferentiatorOutMax=[]  FilterDiffOutCoefMin=[]  FilterDiffOutCoefMax=[]  ReciprocalOutMin=[]  ReciprocalOutMax=[]  SumDenOutMin=[]  SumDenOutMax=[]  SumNumOutMin=[]  SumNumOutMax=[]  DivideOutMin=[]  DivideOutMax=[]  UdiffTsProdOutMin=[]  UdiffTsProdOutMax=[]  NTsProdOutMin=[]  NTsProdOutMax=[]  UintegralTsProdOutMin=[]  UintegralTsProdOutMax=[]  UngainTsProdOutMin=[]  UngainTsProdOutMax=[]  ClampingZeroOutDataTypeStr=Inherit: Inherit via back propagation  ClampingZeroOutMin=[]  ClampingZeroOutMax=[]  FilterDenConstantOutDataTypeStr=Inherit: Inherit via back propagation  FilterDenConstantOutMin=[]  FilterDenConstantOutMax=[]  PCopyOutDataTypeStr=Inherit: Inherit via back propagation  PCopyOutMin=[]  PCopyOutMax=[]  NCopyOutDataTypeStr=Inherit: Inherit via back propagation  NCopyOutMin=[]  NCopyOutMax=[]  IntegratorContinuousStateAttributes=''  IntegratorStateMustResolveToSignalObject=off  IntegratorRTWStateStorageClass=Auto  FilterContinuousStateAttributes=''  FilterStateMustResolveToSignalObject=off  FilterRTWStateStorageClass=Auto  ParallelPVariant=InternalParameters  IdealPVariant=Disabled  IVariant=InternalParameters  DVariant=Disabled  IntegratorVariant=Discrete  SatVariant=Enabled  AWVariant=DiscClampingParallel  PCopyVariant=Disabled  TRVariant=Disabled  FdbkBlocksVariant=Forward  IdealPFdbkVariant=Disabled  SatFdbkVariant=Disabled  DerivativeFilterVariant=Disabled  NVariant=Disabled  NCopyVariant=Disabled_SignalSpec  FilterICVariant=Disabled  IntegratorICVariant=InternalICs  ExternalResetVariant=Disabled  TRSumVariant=Passthrough  SumFdbkVariant=Disabled  SumVariant=Sum_PI  TsampFilterVariant=InternalTs  TsampNgainVariant=Passthrough  TsampIntegralVariant=Disabled_SignalSpec  ExternalSaturationOutDataTypeStr=Inherit: Same as second input  DerivativeSourceVariant=Disabled  PreIntVariant=InternalPreInt
      settings: LibrarySourceBlock=simulink/Discrete/Discrete PID Controller
  id diff : Sum  Inputs=+-
  iq diff : Sum  Inputs=-+
  iq_Ref_gen gain : Gain  Gain=1/PMSM.Kt_peak
  lambda_m : Constant  Value=PMSM.lambda_m
  mag_ref_z2 : UnitDelay  SampleTime=FOC.Ts  HasFrameUpgradeWarning=on
  q-axis current controller : slpidlib/PID Controller  Controller=PI  Form=Parallel  TimeDomain=Discrete-time  UseExternalTs=off  SampleTime=FOC.Ts  IntegratorMethod=Forward Euler  FilterMethod=Forward Euler  ControllerParametersSource=internal  P=FOC.Kp_iq  I=FOC.Ki_iq  UseKiTs=off  D=0  UseExternalDerivativeSource=off  N=100  UseFilter=on  TunerSelectOption=Transfer Function Based (PID Tuner App)  InitialConditionSource=internal  InitialConditionForIntegrator=0  InitialConditionForFilter=0  DifferentiatorICPrevScaledInput=0  ExternalReset=none  TrackingMode=off  Kt=1  LimitOutput=on  SatLimitsSource=internal  UpperSaturationLimit=BAT.V_nom/sqrt(3)  LowerSaturationLimit=-BAT.V_nom/sqrt(3)  LinearizeAsGain=off  AntiWindupMode=clamping  Kb=1  LimitIntegrator=off  UpperIntegratorSaturationLimit=inf  LowerIntegratorSaturationLimit=-inf  POutMin=[]  POutMax=[]  IOutMin=[]  IOutMax=[]  DOutMin=[]  DOutMax=[]  NOutMin=[]  NOutMax=[]  SumOutMin=[]  SumOutMax=[]  SaturationOutMin=[]  SaturationOutMax=[]  PParamMin=[]  PParamMax=[]  IParamMin=[]  IParamMax=[]  DParamMin=[]  DParamMax=[]  NParamMin=[]  NParamMax=[]  KbParamMin=[]  KbParamMax=[]  KtParamMin=[]  KtParamMax=[]  KbOutMin=[]  KbOutMax=[]  KtOutMin=[]  KtOutMax=[]  IntegratorOutMin=[]  IntegratorOutMax=[]  FilterOutMin=[]  FilterOutMax=[]  SumI1OutMin=[]  SumI1OutMax=[]  SumI2OutMin=[]  SumI2OutMax=[]  SumI3OutMin=[]  SumI3OutMax=[]  SumI4OutMin=[]  SumI4OutMax=[]  SumDOutMin=[]  SumDOutMax=[]  DifferentiatorOutMin=[]  DifferentiatorOutMax=[]  FilterDiffOutCoefMin=[]  FilterDiffOutCoefMax=[]  ReciprocalOutMin=[]  ReciprocalOutMax=[]  SumDenOutMin=[]  SumDenOutMax=[]  SumNumOutMin=[]  SumNumOutMax=[]  DivideOutMin=[]  DivideOutMax=[]  UdiffTsProdOutMin=[]  UdiffTsProdOutMax=[]  NTsProdOutMin=[]  NTsProdOutMax=[]  UintegralTsProdOutMin=[]  UintegralTsProdOutMax=[]  UngainTsProdOutMin=[]  UngainTsProdOutMax=[]  ClampingZeroOutDataTypeStr=Inherit: Inherit via back propagation  ClampingZeroOutMin=[]  ClampingZeroOutMax=[]  FilterDenConstantOutDataTypeStr=Inherit: Inherit via back propagation  FilterDenConstantOutMin=[]  FilterDenConstantOutMax=[]  PCopyOutDataTypeStr=Inherit: Inherit via back propagation  PCopyOutMin=[]  PCopyOutMax=[]  NCopyOutDataTypeStr=Inherit: Inherit via back propagation  NCopyOutMin=[]  NCopyOutMax=[]  IntegratorContinuousStateAttributes=''  IntegratorStateMustResolveToSignalObject=off  IntegratorRTWStateStorageClass=Auto  FilterContinuousStateAttributes=''  FilterStateMustResolveToSignalObject=off  FilterRTWStateStorageClass=Auto  ParallelPVariant=InternalParameters  IdealPVariant=Disabled  IVariant=InternalParameters  DVariant=Disabled  IntegratorVariant=Discrete  SatVariant=Enabled  AWVariant=DiscClampingParallel  PCopyVariant=Disabled  TRVariant=Disabled  FdbkBlocksVariant=Forward  IdealPFdbkVariant=Disabled  SatFdbkVariant=Disabled  DerivativeFilterVariant=Disabled  NVariant=Disabled  NCopyVariant=Disabled_SignalSpec  FilterICVariant=Disabled  IntegratorICVariant=InternalICs  ExternalResetVariant=Disabled  TRSumVariant=Passthrough  SumFdbkVariant=Disabled  SumVariant=Sum_PI  TsampFilterVariant=InternalTs  TsampNgainVariant=Passthrough  TsampIntegralVariant=Disabled_SignalSpec  ExternalSaturationOutDataTypeStr=Inherit: Same as second input  DerivativeSourceVariant=Disabled  PreIntVariant=InternalPreInt
      settings: LibrarySourceBlock=simulink/Discrete/Discrete PID Controller
  Vq_g : Outport
  Vd_g : Outport  Port=2
  wires:
  TorqueRef_gen_eff/1 -> iq_Ref_gen gain/1
  iq_Ref_gen gain/1 -> Current Limit to produce iq_ref_gen/1
  id_g/1 -> DQ Decoupling/Feedforward/6(id), id diff/2
  id diff/1 -> d-axis current controller/1
  Current Limit to produce iq_ref_gen/1 -> iq diff/2
  iq diff/1 -> q-axis current controller/1
  iq_g/1 -> iq diff/1, DQ Decoupling/Feedforward/7(iq)
  DQ Limiter/1 -> Vd_g/1
  DQ Limiter/2 -> Vq_g/1
  V_term_B/1 -> Field Weakening/2(V_term), Conversion to V satLim/1
  Conversion to V satLim/1 -> DQ Limiter/3
  Lq/1 -> DQ Decoupling/Feedforward/3(Lq)
  P/1 -> DQ Decoupling/Feedforward/1(p)
  Ld/1 -> DQ Decoupling/Feedforward/2(Ld)
  lambda_m/1 -> DQ Decoupling/Feedforward/4(lambda_m)
  DQ Decoupling/Feedforward/2(vq_cmd) -> DQ Limiter/2
  DQ Decoupling/Feedforward/1(vd_cmd) -> DQ Limiter/1
  q-axis current controller/1 -> DQ Decoupling/Feedforward/8(vq_pi)
  d-axis current controller/1 -> DQ Decoupling/Feedforward/5(vd_pi)
  omega_mech/1 -> DQ Decoupling/Feedforward/9(omega_mech)
  Field Weakening/1(id_ref_fw) -> id diff/1
  DQ Limiter/3 -> mag_ref_z2/1
  mag_ref_z2/1 -> Field Weakening/1(mag_ref)
